simulink model "SimulinkPrado23210715"  (R2023a)
settings: Solver=ode15s  StartTime=0.0  StopTime=10.0  MaxStep=1e-3  RelTol=1e-3
libraries: fl_lib x9, nesl_utility x3, slpidlib x1, simulink x1
settings Model: Creator=LENOVO  LastModifiedBy=IT
settings DataIOCC: SaveOutput=off  SignalLogging=off  DSMLogging=off  ReturnWorkspaceOutputs=off  TimeSaveName=t
settings DebuggingCC: AlgebraicLoopMsg=none  ArtificialAlgebraicLoopMsg=none  MaxConsecutiveZCsMsg=none  ModelReferenceExtraNoncontSigs=none  OperatingPointInterfaceChecksumMismatchMsg=none

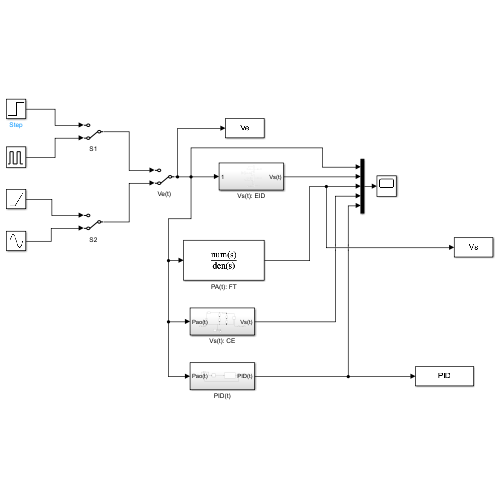
[thumbnail: Simulink's stored preview of the top-level diagram]
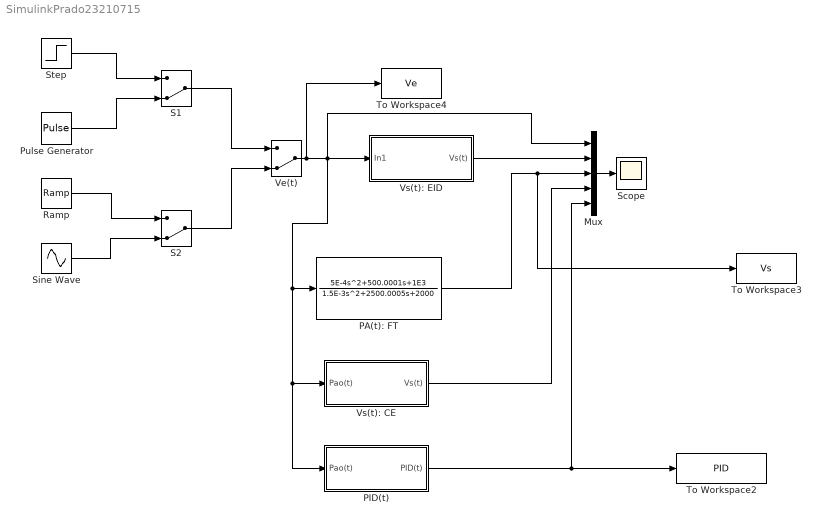
== system SimulinkPrado23210715 ==
  Mux : Mux  Inputs=5
  PA(t): FT : TransferFcn  Numerator=[5E-4, 500.0001, 1E3]  Denominator=[1.5E-3, 2500.0005, 2000]
  PID(t) : Subsystem
  Pulse Generator : DiscretePulseGenerator  PulseType=Time based  Period=10  PulseWidth=10  PhaseDelay=1
  Ramp : simulink/Sources/Ramp  slope=1/10  start=0  InitialOutput=0
  S1 : ManualSwitch  CurrentSetting=0
  S2 : ManualSwitch  CurrentSetting=0
  Scope : Scope
  Sine Wave : Sin  Frequency=pi/2  SampleTime=0
  Step : Step  Time=0  Before=1  SampleTime=0
  To Workspace2 : ToWorkspace  VariableName=PID  SampleTime=-1
  To Workspace3 : ToWorkspace  VariableName=Vs  SampleTime=-1
  To Workspace4 : ToWorkspace  VariableName=Ve  SampleTime=-1
  Ve(t) : ManualSwitch  CurrentSetting=0
  Vs(t): CE : Subsystem
  Vs(t): EID : Subsystem
  wires:
  Vs(t): EID/1(Vs(t)) -> Mux/2
  Mux/1 -> Scope/1
  Step/1 -> S1/1
  Ve(t)/1 -> To Workspace4/1, Mux/1, PID(t)/1(Pao(t)), Vs(t): CE/1(Pao(t)), PA(t): FT/1, Vs(t): EID/1(In1)
  S1/1 -> Ve(t)/1
  Pulse Generator/1 -> S1/2
  S2/1 -> Ve(t)/2
  Ramp/1 -> S2/1
  Sine Wave/1 -> S2/2
  Vs(t): CE/1(Vs(t)) -> Mux/4
  PID(t)/1(PID(t)) -> Mux/5, To Workspace2/1
  PA(t): FT/1 -> To Workspace3/1, Mux/3

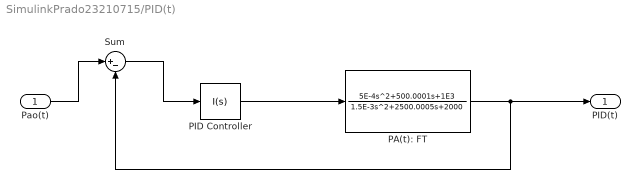
== system SimulinkPrado23210715/PID(t) ==
  Pao(t) : Inport
  PA(t): FT : TransferFcn  Numerator=[5E-4, 500.0001, 1E3]  Denominator=[1.5E-3, 2500.0005, 2000]
  PID Controller : slpidlib/PID Controller  Controller=I  Form=Parallel  TimeDomain=Continuous-time  UseExternalTs=off  SampleTime=-1  IntegratorMethod=Forward Euler  FilterMethod=Forward Euler  ControllerParametersSource=internal  P=0.858862349102461  I=1301.56707675634  UseKiTs=off  D=-0.0392929524714376  N=21.8579234972678  UseFilter=on  TunerSelectOption=Transfer Function Based (PID Tuner App)  InitialConditionSource=internal  InitialConditionForIntegrator=0  InitialConditionForFilter=0  DifferentiatorICPrevScaledInput=0  ExternalReset=none  TrackingMode=off  Kt=1  LimitOutput=off  SatLimitsSource=internal  UpperSaturationLimit=inf  LowerSaturationLimit=-inf  LinearizeAsGain=on  AntiWindupMode=none  Kb=1  LimitIntegrator=off  UpperIntegratorSaturationLimit=inf  LowerIntegratorSaturationLimit=-inf  POutMin=[]  POutMax=[]  IOutMin=[]  IOutMax=[]  DOutMin=[]  DOutMax=[]  NOutMin=[]  NOutMax=[]  SumOutMin=[]  SumOutMax=[]  SaturationOutMin=[]  SaturationOutMax=[]  PParamMin=[]  PParamMax=[]  IParamMin=[]  IParamMax=[]  DParamMin=[]  DParamMax=[]  NParamMin=[]  NParamMax=[]  KbParamMin=[]  KbParamMax=[]  KtParamMin=[]  KtParamMax=[]  KbOutMin=[]  KbOutMax=[]  KtOutMin=[]  KtOutMax=[]  IntegratorOutMin=[]  IntegratorOutMax=[]  FilterOutMin=[]  FilterOutMax=[]  SumI1OutMin=[]  SumI1OutMax=[]  SumI2OutMin=[]  SumI2OutMax=[]  SumI3OutMin=[]  SumI3OutMax=[]  SumI4OutMin=[]  SumI4OutMax=[]  SumDOutMin=[]  SumDOutMax=[]  DifferentiatorOutMin=[]  DifferentiatorOutMax=[]  FilterDiffOutCoefMin=[]  FilterDiffOutCoefMax=[]  ReciprocalOutMin=[]  ReciprocalOutMax=[]  SumDenOutMin=[]  SumDenOutMax=[]  SumNumOutMin=[]  SumNumOutMax=[]  DivideOutMin=[]  DivideOutMax=[]  UdiffTsProdOutMin=[]  UdiffTsProdOutMax=[]  NTsProdOutMin=[]  NTsProdOutMax=[]  UintegralTsProdOutMin=[]  UintegralTsProdOutMax=[]  UngainTsProdOutMin=[]  UngainTsProdOutMax=[]  ClampingZeroOutDataTypeStr=Inherit: Inherit via back propagation  ClampingZeroOutMin=[]  ClampingZeroOutMax=[]  FilterDenConstantOutDataTypeStr=Inherit: Inherit via back propagation  FilterDenConstantOutMin=[]  FilterDenConstantOutMax=[]  PCopyOutDataTypeStr=Inherit: Inherit via back propagation  PCopyOutMin=[]  PCopyOutMax=[]  NCopyOutDataTypeStr=Inherit: Inherit via back propagation  NCopyOutMin=[]  NCopyOutMax=[]  IntegratorContinuousStateAttributes=''  IntegratorStateMustResolveToSignalObject=off  IntegratorRTWStateStorageClass=Auto  FilterContinuousStateAttributes=''  FilterStateMustResolveToSignalObject=off  FilterRTWStateStorageClass=Auto  ParallelPVariant=Disabled  IdealPVariant=Disabled  IVariant=InternalParameters  DVariant=Disabled  IntegratorVariant=Continuous  SatVariant=Disabled  AWVariant=Passthrough  PCopyVariant=Disabled  TRVariant=Disabled  FdbkBlocksVariant=Forward  IdealPFdbkVariant=Disabled  SatFdbkVariant=Disabled  DerivativeFilterVariant=Disabled  NVariant=Disabled  NCopyVariant=Disabled_SignalSpec  FilterICVariant=Disabled  IntegratorICVariant=InternalICs  ExternalResetVariant=Disabled  TRSumVariant=Passthrough  SumFdbkVariant=Disabled  SumVariant=Passthrough_I  TsampFilterVariant=InternalTs  TsampNgainVariant=Passthrough  TsampIntegralVariant=Disabled_SignalSpec  ExternalSaturationOutDataTypeStr=Inherit: Same as second input
  Sum : Sum  Inputs=|+-
  PID(t) : Outport
  wires:
  Pao(t)/1 -> Sum/1
  PA(t): FT/1 -> Sum/2, PID(t)/1
  Sum/1 -> PID Controller/1
  PID Controller/1 -> PA(t): FT/1

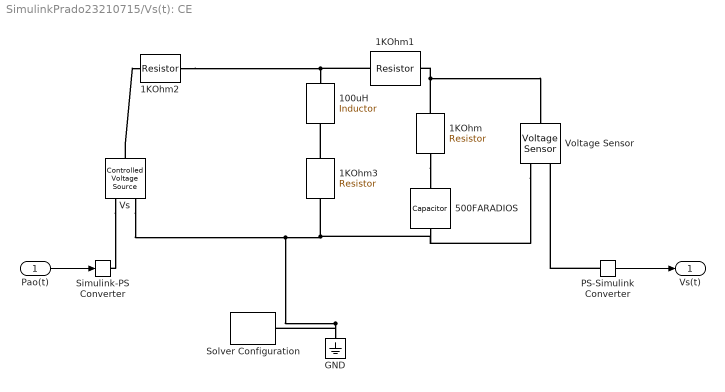
== system SimulinkPrado23210715/Vs(t): CE ==
  Pao(t) : Inport
  100uH : fl_lib/Electrical/Electrical Elements/Inductor  l=100E-6 H  r=0 Ohm  g=1e-9 1/Ohm  i_specify=off  i_priority=None  i=0 A  i_nominal_specify=off  i_nominal_unit=A  i_nominal_value=1  v_specify=off  v_priority=None  v=0 V  v_nominal_specify=off  v_nominal_unit=V  v_nominal_value=1  i_L_specify=off  i_L_priority=High  i_L=0 A  i_L_nominal_specify=off  i_L_nominal_unit=A  i_L_nominal_value=1
  1KOhm{,1..3} (4 alike) : fl_lib/Electrical/Electrical Elements/Resistor  R=1 kOhm  i_specify=off  i_priority=None  i=0 A  i_nominal_specify=off  i_nominal_unit=A  i_nominal_value=1  v_specify=off  v_priority=None  v=0 V  v_nominal_specify=off  v_nominal_unit=V  v_nominal_value=1
  500FARADIOS : fl_lib/Electrical/Electrical Elements/Capacitor  c=500E-6 F  r=1e-6 Ohm  g=0 1/Ohm  i_specify=off  i_priority=None  i=0 A  i_nominal_specify=off  i_nominal_unit=A  i_nominal_value=1  v_specify=off  v_priority=None  v=0 V  v_nominal_specify=off  v_nominal_unit=V  v_nominal_value=1  vc_specify=off  vc_priority=High  vc=0 V  vc_nominal_specify=off  vc_nominal_unit=V  vc_nominal_value=1
  GND : fl_lib/Electrical/Electrical Elements/Electrical Reference
  PS-Simulink Converter : nesl_utility/PS-Simulink Converter  PhysicalDomain=network_engine_domain  SubClassName=ps_output  LeftPortType=input  RightPortType=output  PseudoPeriodic=off  Frequencies=[]  VectorFormat=inherit  Unit=inherit  AffineConversion=off
  Simulink-PS Converter : nesl_utility/Simulink-PS Converter  PhysicalDomain=network_engine_domain  SubClassName=ps_input  LeftPortType=input  RightPortType=output  PseudoPeriodic=off  Frequencies=[]  NoiseDistribution=none  NoiseParameters=[]  Unit=1  AffineConversion=off  FilteringAndDerivatives=provide  SimscapeFilterOrder=1  InputFilterTimeConstant=0.001  UdotUserProvided=0
  Solver Configuration : nesl_utility/Solver Configuration  PhysicalDomain=network_engine_domain  SubClassName=solver  LeftPortType=input  RightPortType=generic  Tones=[]  Harmonics=[]  SimulateNoise=off  Profile=off  UseLocalSampling=off  EnableSwitchedLinearOptims=on  FrequencyDomain=off  UseCCode=off  RelTol=0.001  AbsTol=0.001  MinStep=1e-09  ToWorkspace=off  RevertToSquareIcSolve=off  NumHomotopyIterations=100  PhasorMode=off  PhasorModeNumHarmonics=1  ConsistencySolver=NEWTON_XTOL_AFTER_FTOL  IndexReductionMethod=DerivativeReplacement  DoDC=off  ResidualTolerance=1e-09  ConsistencyTolSource=GLOBAL  ConsistencyAbsTol=0.001  ConsistencyRelTol=0.001  ConsistencyTolFactor=0.001  UseLocalSolver=off  LocalSolverChoice=NE_BACKWARD_EULER_ADVANCER  ResolveIndetEquations=on  FunctionEvalNumThread=1  LocalSolverSampleTime=0.001  DoFixedCost=off  MaxNonlinIter=3  MaxModeIter=2  ComputeImpulses=off  ImpulseIterations=2  LinearAlgebra=auto  LinearAlgebraNumThread=0  EquationFormulation=NE_TIME_EF  DelaysMemoryBudget=1024  AutomaticFiltering=on  FilteringTimeConstant=0.001  PartitionStorageMethod=AS_NEEDED  PartitionMemoryBudget=1024  PartitionMethod=ROBUST
  Voltage Sensor : fl_lib/Electrical/Electrical Sensors/Voltage Sensor
  Vs : fl_lib/Electrical/Electrical Sources/Controlled Voltage Source
  Vs(t) : Outport
  wires:
  Pao(t)/1 -> Simulink-PS Converter/1
  PS-Simulink Converter/1 -> Vs(t)/1
  connections:
  Vs/RConn2 -- Voltage Sensor/RConn2 -- 500FARADIOS/RConn1 -- 1KOhm3/RConn1 -- Solver Configuration/RConn1 -- GND/LConn1
  Vs/LConn1 -- 1KOhm2/LConn1
  Vs/RConn1 -- Simulink-PS Converter/RConn1
  1KOhm2/RConn1 -- 1KOhm1/RConn1 -- 100uH/LConn1
  1KOhm/LConn1 -- Voltage Sensor/LConn1 -- 1KOhm1/LConn1
  1KOhm/RConn1 -- 500FARADIOS/LConn1
  PS-Simulink Converter/LConn1 -- Voltage Sensor/RConn1
  1KOhm3/LConn1 -- 100uH/RConn1

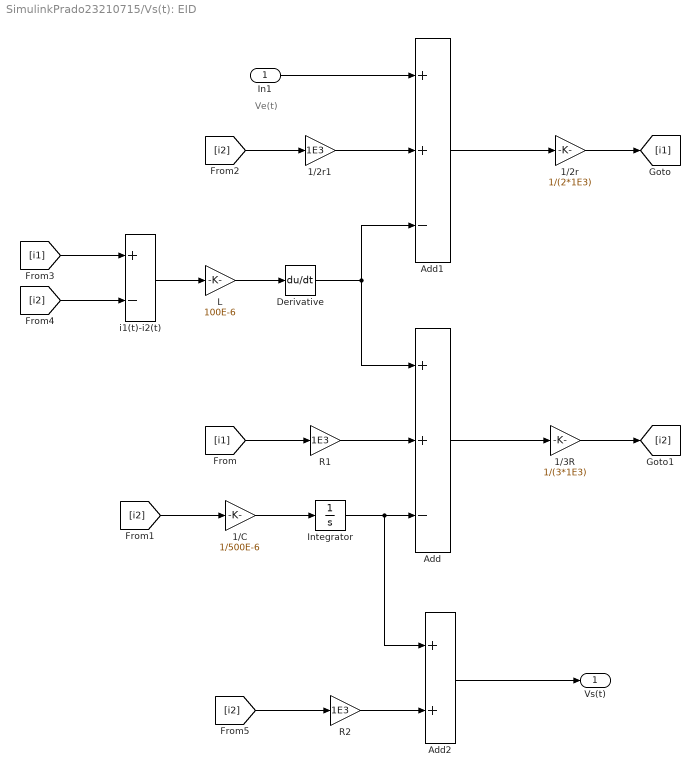
== system SimulinkPrado23210715/Vs(t): EID ==
  note: Ve(t)
  In1 : Inport
  1/2r : Gain  Gain=1/(2*1E3)
  1/2r1 : Gain  Gain=1E3
  1/3R : Gain  Gain=1/(3*1E3)
  1/C : Gain  Gain=1/500E-6
  Add : Sum  Inputs=++-
  Add1 : Sum  Inputs=++-
  Add2 : Sum
  Derivative : Derivative
  Integrator : Integrator
  L : Gain  Gain=100E-6
  R1 : Gain  Gain=1E3
  R2 : Gain  Gain=1E3
  i1(t)-i2(t) : Sum  Inputs=+-
  Vs(t) : Outport
  wires:
  Add1/1 -> 1/2r/1
  Add/1 -> 1/3R/1
  1/2r/1 -> [i1]
  1/2r1/1 -> Add1/2
  [i2] -> 1/2r1/1
  Derivative/1 -> Add1/3, Add/1
  L/1 -> Derivative/1
  i1(t)-i2(t)/1 -> L/1
  [i1] -> i1(t)-i2(t)/1
  [i2] -> i1(t)-i2(t)/2
  R1/1 -> Add/2
  In1/1 -> Add1/1
  [i1] -> R1/1
  Integrator/1 -> Add2/1, Add/3
  1/C/1 -> Integrator/1
  [i2] -> 1/C/1
  Add2/1 -> Vs(t)/1
  R2/1 -> Add2/2
  [i2] -> R2/1
  1/3R/1 -> [i2]
